simulink model "gm_sampleModel1636_4_sub"  (R2023a)
settings: Solver=VariableStepAuto  StartTime=0.0  StopTime=10.0  RelTol=1e-3
libraries: hdlsllib x4, simulink x1
settings Model: Creator=user1  LastModifiedBy=user1
settings OptimizationCC: BlockReduction=off  ConditionallyExecuteInputs=off
settings DebuggingCC: InheritedTsInSrcMsg=none

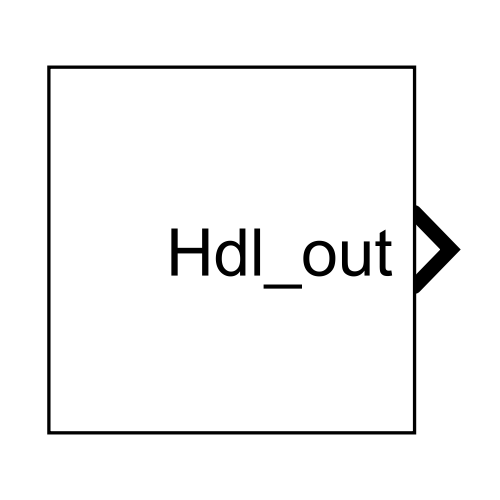
[thumbnail: Simulink's stored preview of the top-level diagram]
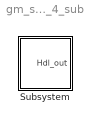
== system gm_sampleModel1636_4_sub ==
  Subsystem : Subsystem

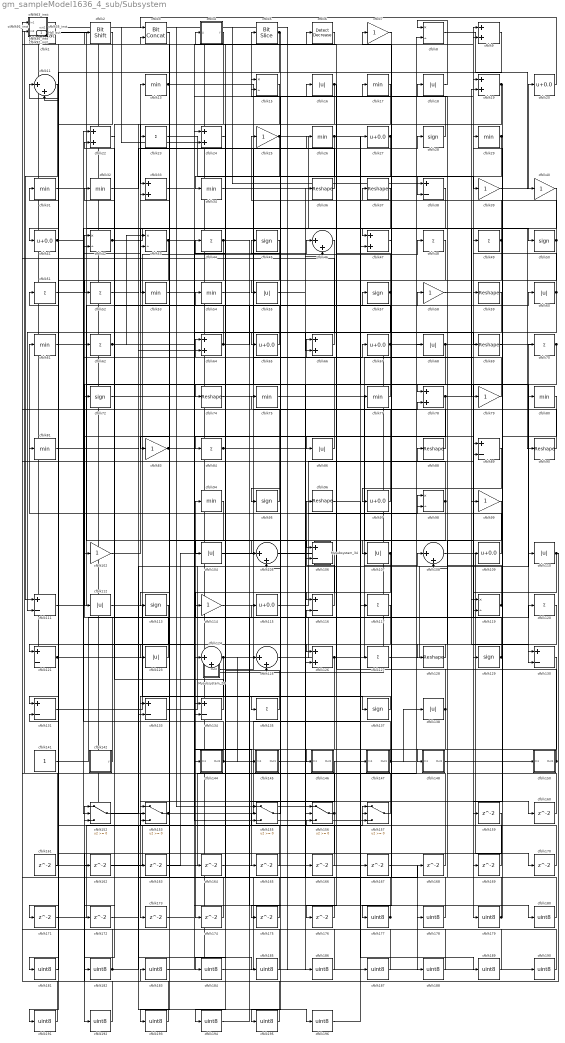
== system gm_sampleModel1636_4_sub/Subsystem ==
  Mysubsystem_20 : Subsystem
  Mysubsystem_34 : Subsystem
  cfblk1 : hdlsllib/Logic and Bit Operations/Bit Concat  numInputs=2
  cfblk101_inst : Subsystem
  cfblk{7,25,39..40,58,79,83,99,102,114} (10 alike) : Gain  OutDataTypeStr=uint8
  cfblk{16,18,55,60,68,86,104,107,110,112,123,138} (12 alike) : Abs  OutDataTypeStr=uint8  SaturateOnIntegerOverflow=off
  cfblk{11,46,105,108,124..125} (6 alike) : Sum  Inputs=|++  OutDataTypeStr=uint8
  cfblk{38,89,106,111,116,121,130..131,133..134} (10 alike) : Sum  Inputs=+-  OutDataTypeStr=uint8
  cfblk{20,27,41,65,67,97,109,115} (8 alike) : Bias  Bias=0.0  SaturateOnIntegerOverflow=off
  cfblk{28,45,50,57,72,95,113,129,137} (9 alike) : Signum
  cfblk{23,44,48..49,51..52,62,70,84,117,120,127,135} (13 alike) : Sum  Inputs=+  OutDataTypeStr=uint8
  cfblk{8,15,42..43,98,119} (6 alike) : Product  Inputs=*/  OutDataTypeStr=uint8  RndMeth=Zero  SaturateOnIntegerOverflow=on
  cfblk122_inst : Subsystem
  cfblk{9,19,22,24,33,47,64,66,78,126} (10 alike) : Sum  OutDataTypeStr=uint8
  cfblk{36..37,59,69,74,88,90,96,128} (9 alike) : Reshape
  cfblk12_inst : Subsystem
  cfblk{13,17,26,29,31..32,34,53..54,61,75,77,80..81,94} (15 alike) : MinMax  OutDataTypeStr=uint8
  cfblk141 : Constant  OutDataTypeStr=uint8  SampleTime=-1
  cfblk142 : Subsystem  mask(Counter Free-Running){NumBits=double(16), tsamp=double(-1)}
      mask prompts: NumBits "Simulink:masks:NumberOfBits_MP"; tsamp "Simulink:masks:SampleTime_MP"
      mask help: Simulink:masks:CounterFreeRunning_MD
  cfblk144 : Subsystem
  cfblk145 : Subsystem
  cfblk146 : Subsystem
  cfblk147 : Subsystem
  cfblk148 : Subsystem
  cfblk150 : Subsystem
  cfblk{152..153,155..157} (5 alike) : Switch  OutDataTypeStr=uint8  SaturateOnIntegerOverflow=off  InputSameDT=off
  cfblk{159..176} (18 alike) : Delay  SampleTime=1
  cfblk{177..196} (20 alike) : DataTypeConversion  OutDataTypeStr=uint8  SaturateOnIntegerOverflow=off  RndMeth=Floor
  cfblk2 : hdlsllib/Logic and Bit Operations/Bit Shift  mode=Shift Left Logical  N=0
  cfblk3 : hdlsllib/Logic and Bit Operations/Bit Concat  numInputs=2
  cfblk30_inst : Subsystem
  cfblk35_inst : Subsystem
  cfblk4 : Subsystem  mask(Detect Rise Nonnegative){vinit=double(0), InputProcessing=Elements as channels (sample based), OutDataTypeStr=uint8}
      mask prompts: vinit "Simulink:masks:InitialCondition_MP"; InputProcessing "Simulink:masks:InputProcessing_MP"; OutDataTypeStr "Simulink:masks:OutputDataType_MP"
      mask help: Simulink:masks:DetectRiseNonnegative_MD
      mask init:
      | InputProcessing = 'Elements as channels (sample based)';
      | OutDataTypeStr = 'uint8';
      | vinit = double(0);
      mask TypeOptions InputProcessing: Simulink:masks:ColumnsAsChannelsFrameBased | Simulink:masks:ElementsAsChannelsSampleBased
      mask TypeOptions OutDataTypeStr: Simulink:masks:uint8 | Simulink:masks:boolean
      mask Display: fprintf('U >= 0\n&  NOT\nU/z >= 0')
  cfblk5 : hdlsllib/Logic and Bit Operations/Bit Slice  lidx=7  ridx=0
  cfblk6 : simulink/Logic and Bit Operations/Detect Decrease  vinit=0.0  OutDataTypeStr=uint8
      settings: LibrarySourceBlock=|
      | hdlsllib/Logic and Bit
      | Operations/Detect
      | Decrease
  cfblk63_inst : Subsystem
  cfblk91_inst : Subsystem
  cfblk92_inst : Subsystem
  Hdl_out : Outport  OutDataTypeStr=uint8  SampleTime=1
  wires:
  Mysubsystem_20/1(Out2) -> cfblk78/2
  Mysubsystem_34/1(Out1) -> cfblk161/1
  cfblk1/1 -> cfblk179/1
  cfblk101_inst/1(out1) -> cfblk190/1
  cfblk102/1 -> cfblk13/1
  cfblk104/1 -> cfblk67/1
  cfblk105/1 -> cfblk88/1
  cfblk106/1 -> cfblk174/1
  cfblk107/1 -> cfblk134/2, cfblk144/1(In1)
  cfblk108/1 -> cfblk170/1
  cfblk109/1 -> cfblk61/1
  cfblk11/1 -> cfblk111/1
  cfblk110/1 -> cfblk183/1, cfblk169/1
  cfblk111/1 -> cfblk54/1
  cfblk112/1 -> cfblk135/1
  cfblk113/1 -> cfblk191/1
  cfblk114/1 -> cfblk28/1
  cfblk115/1 -> cfblk98/1
  cfblk116/1 -> cfblk96/1
  cfblk117/1 -> cfblk195/1
  cfblk119/1 -> cfblk66/1, cfblk75/1
  cfblk12_inst/1(out1) -> cfblk187/1
  cfblk120/1 -> cfblk193/1
  cfblk121/1 -> cfblk137/1, cfblk48/1
  cfblk122_inst/1(out1) -> cfblk156/1, cfblk167/1
  cfblk123/1 -> cfblk42/1
  cfblk124/1 -> cfblk116/2, cfblk173/1
  cfblk125/1 -> cfblk68/1
  cfblk126/1 -> cfblk9/1, cfblk184/1, cfblk108/1
  cfblk127/1 -> cfblk70/1
  cfblk128/1 -> cfblk121/1
  cfblk129/1 -> cfblk59/1, cfblk94/1
  cfblk13/1 -> cfblk130/2, cfblk166/1
  cfblk130/1 -> cfblk148/1(In1)
  cfblk131/1 -> cfblk58/1
  cfblk133/1 -> cfblk110/1
  cfblk134/1 -> cfblk22/2
  cfblk135/1 -> cfblk44/1
  cfblk137/1 -> cfblk133/1
  cfblk138/1 -> cfblk165/1, cfblk6/1
  cfblk141/1 -> cfblk27/1
  cfblk142/1(y) -> cfblk42/2
  cfblk144/1(Out1) -> cfblk22/1, cfblk125/1
  cfblk145/1(Out1) -> cfblk186/1
  cfblk146/1(Out1) -> cfblk153/1
  cfblk147/1(Out1) -> cfblk89/2, cfblk138/1, cfblk4/1(U)
  cfblk148/1(Out1) -> cfblk150/1(In1)
  cfblk15/1 -> cfblk33/1
  cfblk150/1(Out1) -> cfblk37/1, cfblk17/1
  cfblk152/1 -> Mysubsystem_34/1(In1)
  cfblk153/1 -> cfblk47/2, Hdl_out/1
  cfblk155/1 -> cfblk115/1
  cfblk156/1 -> cfblk192/1, cfblk31/1
  cfblk157/1 -> cfblk45/1
  cfblk159/1 -> cfblk181/1
  cfblk16/1 -> cfblk65/1, cfblk133/2, cfblk126/1
  cfblk160/1 -> cfblk98/2
  cfblk161/1 -> cfblk91_inst/2(in2)
  cfblk162/1 -> cfblk155/2
  cfblk163/1 -> cfblk8/2
  cfblk164/1 -> cfblk157/1
  cfblk165/1 -> cfblk153/2
  cfblk166/1 -> cfblk155/1
  cfblk167/1 -> cfblk188/1
  cfblk168/1 -> cfblk63_inst/2(in2)
  cfblk169/1 -> cfblk156/3
  cfblk17/1 -> cfblk84/1
  cfblk170/1 -> cfblk11/1
  cfblk171/1 -> cfblk153/3
  cfblk172/1 -> cfblk157/2
  cfblk173/1 -> cfblk180/1
  cfblk174/1 -> cfblk134/1
  cfblk175/1 -> cfblk131/2
  cfblk176/1 -> cfblk64/1
  cfblk177/1 -> cfblk63_inst/1(in1), cfblk3/2
  cfblk178/1 -> cfblk7/1
  cfblk179/1 -> cfblk108/2, cfblk49/1
  cfblk18/1 -> cfblk8/1
  cfblk180/1 -> cfblk1/1
  cfblk181/1 -> cfblk1/2
  cfblk182/1 -> cfblk92_inst/1(in1), cfblk168/1
  cfblk183/1 -> cfblk46/1
  cfblk184/1 -> cfblk46/2
  cfblk185/1 -> cfblk122_inst/1(in1)
  cfblk186/1 -> cfblk81/1
  cfblk187/1 -> cfblk122_inst/2(in2)
  cfblk188/1 -> cfblk12_inst/1(in1)
  cfblk189/1 -> cfblk12_inst/2(in2)
  cfblk19/1 -> cfblk106/1, cfblk119/2
  cfblk190/1 -> cfblk152/1
  cfblk191/1 -> cfblk101_inst/1(in1)
  cfblk192/1 -> cfblk101_inst/2(in2)
  cfblk193/1 -> cfblk152/3
  cfblk194/1 -> cfblk120/1
  cfblk195/1 -> cfblk91_inst/1(in1)
  cfblk196/1 -> cfblk117/1
  cfblk2/1 -> cfblk41/1
  cfblk20/1 -> cfblk3/1
  cfblk22/1 -> cfblk52/1
  cfblk23/1 -> cfblk39/1
  cfblk24/1 -> cfblk74/1
  cfblk25/1 -> cfblk119/1, cfblk34/1
  cfblk26/1 -> cfblk78/1, cfblk175/1
  cfblk27/1 -> cfblk47/1, cfblk105/1
  cfblk28/1 -> cfblk5/1
  cfblk29/1 -> cfblk38/2, cfblk116/1
  cfblk3/1 -> cfblk113/1
  cfblk30_inst/1(out1) -> cfblk24/2
  cfblk31/1 -> cfblk99/1
  cfblk32/1 -> cfblk26/1
  cfblk33/1 -> cfblk19/1
  cfblk34/1 -> cfblk90/1
  cfblk35_inst/1(out1) -> cfblk121/2, cfblk127/1
  cfblk36/1 -> cfblk23/1
  cfblk37/1 -> cfblk172/1
  cfblk38/1 -> cfblk152/2
  cfblk39/1 -> cfblk20/1
  cfblk4/1(Y) -> cfblk162/1
  cfblk40/1 -> cfblk53/1
  cfblk41/1 -> cfblk86/1, cfblk43/2
  cfblk42/1 -> cfblk50/1, cfblk196/1
  cfblk43/1 -> cfblk69/1, cfblk131/1
  cfblk44/1 -> cfblk156/2, cfblk83/1
  cfblk45/1 -> cfblk123/1
  cfblk46/1 -> cfblk182/1
  cfblk47/1 -> cfblk107/1
  cfblk48/1 -> cfblk194/1
  cfblk49/1 -> cfblk25/1, cfblk146/1(In1)
  cfblk5/1 -> cfblk95/1, cfblk11/2
  cfblk50/1 -> cfblk55/1, cfblk16/1, cfblk15/1
  cfblk51/1 -> cfblk124/1
  cfblk52/1 -> cfblk64/2
  cfblk53/1 -> cfblk155/3
  cfblk54/1 -> cfblk178/1
  cfblk55/1 -> cfblk36/1
  cfblk57/1 -> cfblk2/1, cfblk125/2, cfblk111/2
  cfblk58/1 -> cfblk79/1
  cfblk59/1 -> cfblk164/1
  cfblk6/1 -> cfblk92_inst/2(in2)
  cfblk60/1 -> cfblk66/2, cfblk29/1
  cfblk61/1 -> cfblk106/2
  cfblk62/1 -> cfblk89/1, cfblk43/1
  cfblk63_inst/1(out1) -> cfblk157/3
  cfblk64/1 -> cfblk57/1, cfblk33/2
  cfblk65/1 -> cfblk32/1
  cfblk66/1 -> cfblk30_inst/2(in2)
  cfblk67/1 -> cfblk112/1, cfblk15/2
  cfblk68/1 -> cfblk105/2, cfblk176/1
  cfblk69/1 -> cfblk159/1
  cfblk7/1 -> cfblk177/1
  cfblk70/1 -> cfblk124/2, cfblk102/1
  cfblk72/1 -> cfblk80/1
  cfblk74/1 -> cfblk160/1
  cfblk75/1 -> cfblk109/1
  cfblk77/1 -> cfblk72/1
  cfblk78/1 -> cfblk19/2, cfblk130/1, cfblk104/1
  cfblk79/1 -> cfblk18/1
  cfblk8/1 -> cfblk40/1
  cfblk80/1 -> cfblk129/1
  cfblk81/1 -> cfblk185/1
  cfblk83/1 -> cfblk9/2, cfblk145/1(In1)
  cfblk84/1 -> cfblk60/1, cfblk126/2
  cfblk86/1 -> cfblk62/1
  cfblk88/1 -> cfblk24/1
  cfblk89/1 -> cfblk97/1
  cfblk9/1 -> cfblk171/1
  cfblk90/1 -> cfblk51/1
  cfblk91_inst/1(out1) -> cfblk38/1, cfblk147/1(In1)
  cfblk92_inst/1(out1) -> cfblk77/1
  cfblk94/1 -> cfblk163/1
  cfblk95/1 -> cfblk30_inst/1(in1)
  cfblk96/1 -> cfblk189/1
  cfblk97/1 -> cfblk35_inst/1(in1)
  cfblk98/1 -> cfblk35_inst/2(in2), cfblk114/1
  cfblk99/1 -> cfblk128/1

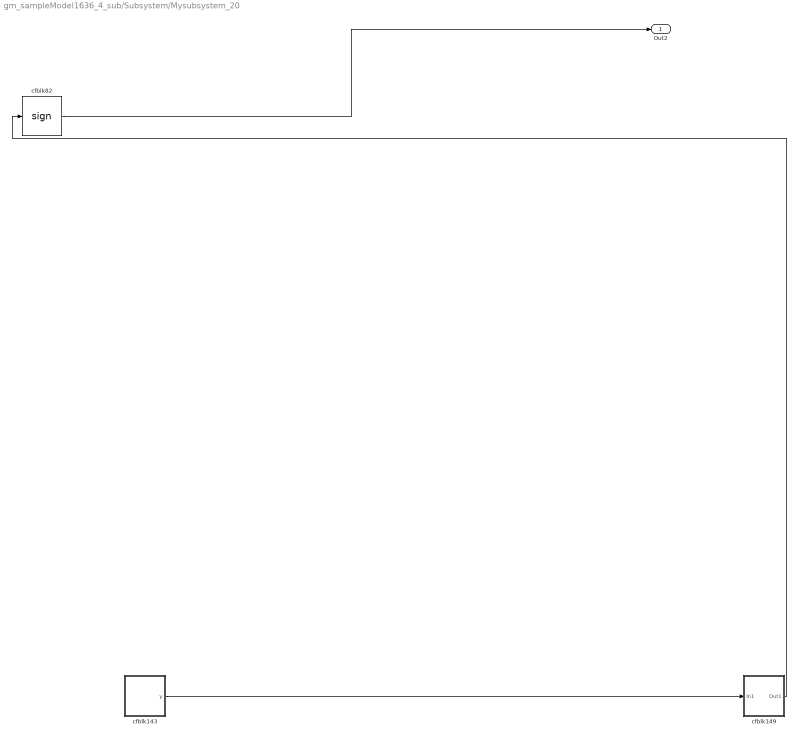
== system gm_sampleModel1636_4_sub/Subsystem/Mysubsystem_20 ==
  cfblk143 : Subsystem  mask(Counter Limited){uplimit=double(7), tsamp=double(-1)}
      mask prompts: uplimit "Simulink:masks:UpperLimit_MP"; tsamp "Simulink:masks:SampleTime_MP"
      mask help: Simulink:masks:CounterLimited_MD
      mask init:
      | nbits = double(8);
      | tsamp = double(-1);
      | uplimit = double(7);
  cfblk149 : Subsystem
  cfblk82 : Signum
  Out2 : Outport  SampleTime=1
  wires:
  cfblk143/1(y) -> cfblk149/1(In1)
  cfblk149/1(Out1) -> cfblk82/1
  cfblk82/1 -> Out2/1

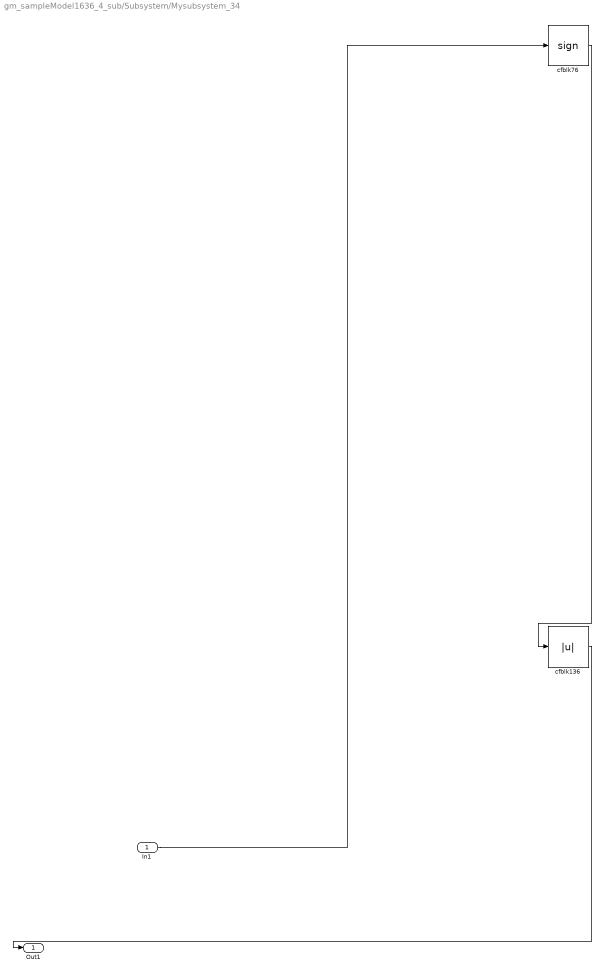
== system gm_sampleModel1636_4_sub/Subsystem/Mysubsystem_34 ==
  In1 : Inport  OutDataTypeStr=uint8  PortDimensions=1  SampleTime=1
  cfblk136 : Abs  SaturateOnIntegerOverflow=off
  cfblk76 : Signum
  Out1 : Outport  SampleTime=1
  wires:
  In1/1 -> cfblk76/1
  cfblk136/1 -> Out1/1
  cfblk76/1 -> cfblk136/1

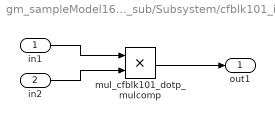
== system gm_sampleModel1636_4_sub/Subsystem/cfblk101_inst ==
  in1 : Inport  OutDataTypeStr=uint8  SampleTime=1
  in2 : Inport  Port=2  OutDataTypeStr=uint8  SampleTime=1
  mul_cfblk101_dotp_mulcomp : Product  Inputs=**  OutDataTypeStr=uint8  SampleTime=1
  out1 : Outport  OutDataTypeStr=uint8  SampleTime=1
  wires:
  in1/1 -> mul_cfblk101_dotp_mulcomp/1
  in2/1 -> mul_cfblk101_dotp_mulcomp/2
  mul_cfblk101_dotp_mulcomp/1 -> out1/1

== system gm_sampleModel1636_4_sub/Subsystem/cfblk122_inst ==
  in1 : Inport  OutDataTypeStr=uint8  SampleTime=1
  in2 : Inport  Port=2  OutDataTypeStr=uint8  SampleTime=1
  mul_cfblk122_dotp_mulcomp : Product  Inputs=**  OutDataTypeStr=uint8  SampleTime=1
  out1 : Outport  OutDataTypeStr=uint8  SampleTime=1
  wires:
  in1/1 -> mul_cfblk122_dotp_mulcomp/1
  in2/1 -> mul_cfblk122_dotp_mulcomp/2
  mul_cfblk122_dotp_mulcomp/1 -> out1/1

== system gm_sampleModel1636_4_sub/Subsystem/cfblk12_inst ==
  in1 : Inport  OutDataTypeStr=uint8  SampleTime=1
  in2 : Inport  Port=2  OutDataTypeStr=uint8  SampleTime=1
  mul_cfblk12_dotp_mulcomp : Product  Inputs=**  OutDataTypeStr=uint8  SampleTime=1
  out1 : Outport  OutDataTypeStr=uint8  SampleTime=1
  wires:
  in1/1 -> mul_cfblk12_dotp_mulcomp/1
  in2/1 -> mul_cfblk12_dotp_mulcomp/2
  mul_cfblk12_dotp_mulcomp/1 -> out1/1

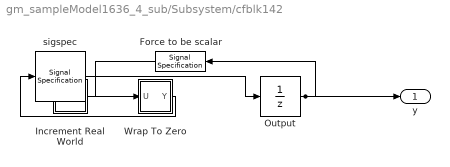
== system gm_sampleModel1636_4_sub/Subsystem/cfblk142 ==
  Force to be scalar : SignalSpecification  DisableCoverage=on  Dimensions=1
  Increment Real World : Subsystem  mask(Real World Value Increment){}
      mask help: Simulink:masks:RealWorldValueIncrement_MD
      mask Display: disp('V++')
  Output : UnitDelay  InitialCondition=0.0  SampleTime=tsamp  HasFrameUpgradeWarning=on
  Wrap To Zero : Subsystem  mask(Wrap To Zero){Threshold=double(65535)}
      mask prompts: Threshold "Simulink:masks:Threshold_MP"
      mask help: Simulink:masks:WrapToZero_MD
  sigspec : SignalSpecification  OutDataTypeStr=uint16  Dimensions=1
  y : Outport  SampleTime=1
  wires:
  Force to be scalar/1 -> Increment Real World/1(u)
  Increment Real World/1(y) -> Wrap To Zero/1(U)
  Output/1 -> Force to be scalar/1, y/1
  Wrap To Zero/1(Y) -> sigspec/1
  sigspec/1 -> Output/1

== system gm_sampleModel1636_4_sub/Subsystem/cfblk144 ==
  In1 : Inport  OutDataTypeStr=uint8  PortDimensions=1  SampleTime=1
  Out1 : Outport  SampleTime=1
  wires:
  In1/1 -> Out1/1

== system gm_sampleModel1636_4_sub/Subsystem/cfblk145 ==
  In1 : Inport  OutDataTypeStr=uint8  PortDimensions=1  SampleTime=1
  Out1 : Outport  SampleTime=1
  wires:
  In1/1 -> Out1/1

== system gm_sampleModel1636_4_sub/Subsystem/cfblk146 ==
  In1 : Inport  OutDataTypeStr=uint8  PortDimensions=1  SampleTime=1
  Out1 : Outport  SampleTime=1
  wires:
  In1/1 -> Out1/1

== system gm_sampleModel1636_4_sub/Subsystem/cfblk147 ==
  In1 : Inport  OutDataTypeStr=uint8  PortDimensions=1  SampleTime=1
  Out1 : Outport  SampleTime=1
  wires:
  In1/1 -> Out1/1

== system gm_sampleModel1636_4_sub/Subsystem/cfblk148 ==
  In1 : Inport  OutDataTypeStr=uint8  PortDimensions=1  SampleTime=1
  Out1 : Outport  SampleTime=1
  wires:
  In1/1 -> Out1/1

== system gm_sampleModel1636_4_sub/Subsystem/cfblk150 ==
  In1 : Inport  OutDataTypeStr=uint8  PortDimensions=1  SampleTime=1
  Out1 : Outport  SampleTime=1
  wires:
  In1/1 -> Out1/1

== system gm_sampleModel1636_4_sub/Subsystem/cfblk30_inst ==
  in1 : Inport  OutDataTypeStr=uint8  SampleTime=1
  in2 : Inport  Port=2  OutDataTypeStr=uint8  SampleTime=1
  mul_cfblk30_dotp_mulcomp : Product  Inputs=**  OutDataTypeStr=uint8  SampleTime=1
  out1 : Outport  OutDataTypeStr=uint8  SampleTime=1
  wires:
  in1/1 -> mul_cfblk30_dotp_mulcomp/1
  in2/1 -> mul_cfblk30_dotp_mulcomp/2
  mul_cfblk30_dotp_mulcomp/1 -> out1/1

== system gm_sampleModel1636_4_sub/Subsystem/cfblk35_inst ==
  in1 : Inport  OutDataTypeStr=uint8  SampleTime=1
  in2 : Inport  Port=2  OutDataTypeStr=uint8  SampleTime=1
  mul_cfblk35_dotp_mulcomp : Product  Inputs=**  OutDataTypeStr=uint8  SampleTime=1
  out1 : Outport  OutDataTypeStr=uint8  SampleTime=1
  wires:
  in1/1 -> mul_cfblk35_dotp_mulcomp/1
  in2/1 -> mul_cfblk35_dotp_mulcomp/2
  mul_cfblk35_dotp_mulcomp/1 -> out1/1

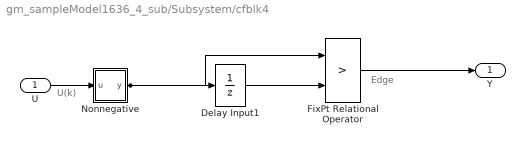
== system gm_sampleModel1636_4_sub/Subsystem/cfblk4 ==
  note: U(k)
  note: Edge
  U : Inport  OutDataTypeStr=uint8  SampleTime=1
  Delay Input1 : UnitDelay  Description=Store in Global RAM  DisableCoverage=on  InitialCondition=vinit  SampleTime=-1  HasFrameUpgradeWarning=on
  FixPt Relational Operator : RelationalOperator  Operator=>  OutDataTypeStr=fixdt(0, 8)  ZeroCross=off  InputSameDT=off
  Nonnegative : Subsystem  mask(Compare To Zero){relop=>=, OutDataTypeStr=boolean, ZeroCross=off}
      mask prompts: relop "Simulink:masks:Operator_MP"; OutDataTypeStr "Simulink:masks:OutputDataType_MP"; ZeroCross "Simulink:masks:EnableZerocrossingDetection_MP"
      mask help: Simulink:masks:CompareToZero_MD
      mask init:
      | OutDataTypeStr = 'boolean';
      | ZeroCross = 'off';
      | blkName = 'sampleModel1636_4_sub/Subsystem/cfblk4/Nonnegative';
      | relop = '>=';
      | setValue = 'boolean';
      mask TypeOptions relop: == | ~= | < | <= | >= | >
      mask TypeOptions OutDataTypeStr: Simulink:masks:uint8 | Simulink:masks:boolean
      mask Callback ZeroCross: sl('zeroCrossEnable', gcbh);
      mask Display: disp([relop,' 0'])
  Y : Outport  SampleTime=1
  wires:
  U/1 -> Nonnegative/1(u)
  Delay Input1/1 -> FixPt Relational Operator/2
  FixPt Relational Operator/1 -> Y/1
  Nonnegative/1(y) -> FixPt Relational Operator/1, Delay Input1/1

== system gm_sampleModel1636_4_sub/Subsystem/cfblk63_inst ==
  in1 : Inport  OutDataTypeStr=uint8  SampleTime=1
  in2 : Inport  Port=2  OutDataTypeStr=uint8  SampleTime=1
  mul_cfblk63_dotp_mulcomp : Product  Inputs=**  OutDataTypeStr=uint8  SampleTime=1
  out1 : Outport  OutDataTypeStr=uint8  SampleTime=1
  wires:
  in1/1 -> mul_cfblk63_dotp_mulcomp/1
  in2/1 -> mul_cfblk63_dotp_mulcomp/2
  mul_cfblk63_dotp_mulcomp/1 -> out1/1

== system gm_sampleModel1636_4_sub/Subsystem/cfblk91_inst ==
  in1 : Inport  OutDataTypeStr=uint8  SampleTime=1
  in2 : Inport  Port=2  OutDataTypeStr=uint8  SampleTime=1
  mul_cfblk91_dotp_mulcomp : Product  Inputs=**  OutDataTypeStr=uint8  SampleTime=1
  out1 : Outport  OutDataTypeStr=uint8  SampleTime=1
  wires:
  in1/1 -> mul_cfblk91_dotp_mulcomp/1
  in2/1 -> mul_cfblk91_dotp_mulcomp/2
  mul_cfblk91_dotp_mulcomp/1 -> out1/1

== system gm_sampleModel1636_4_sub/Subsystem/cfblk92_inst ==
  in1 : Inport  OutDataTypeStr=uint8  SampleTime=1
  in2 : Inport  Port=2  OutDataTypeStr=uint8  SampleTime=1
  mul_cfblk92_dotp_mulcomp : Product  Inputs=**  OutDataTypeStr=uint8  SampleTime=1
  out1 : Outport  OutDataTypeStr=uint8  SampleTime=1
  wires:
  in1/1 -> mul_cfblk92_dotp_mulcomp/1
  in2/1 -> mul_cfblk92_dotp_mulcomp/2
  mul_cfblk92_dotp_mulcomp/1 -> out1/1

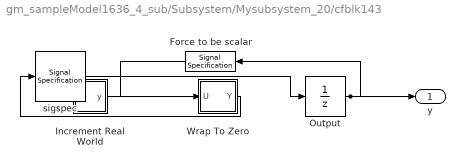
== system gm_sampleModel1636_4_sub/Subsystem/Mysubsystem_20/cfblk143 ==
  Force to be scalar : SignalSpecification  DisableCoverage=on  Dimensions=1
  Increment Real World : Subsystem  mask(Real World Value Increment){}
      mask help: Simulink:masks:RealWorldValueIncrement_MD
      mask Display: disp('V++')
  Output : UnitDelay  InitialCondition=0.0  SampleTime=tsamp  HasFrameUpgradeWarning=on
  Wrap To Zero : Subsystem  mask(Wrap To Zero){Threshold=double(7)}
      mask prompts: Threshold "Simulink:masks:Threshold_MP"
      mask help: Simulink:masks:WrapToZero_MD
  sigspec : SignalSpecification  OutDataTypeStr=uint8  Dimensions=1
  y : Outport  SampleTime=1
  wires:
  Force to be scalar/1 -> Increment Real World/1(u)
  Increment Real World/1(y) -> Wrap To Zero/1(U)
  Output/1 -> Force to be scalar/1, y/1
  Wrap To Zero/1(Y) -> sigspec/1
  sigspec/1 -> Output/1

== system gm_sampleModel1636_4_sub/Subsystem/Mysubsystem_20/cfblk149 ==
  In1 : Inport  OutDataTypeStr=uint8  PortDimensions=1  SampleTime=1
  Out1 : Outport  SampleTime=1
  wires:
  In1/1 -> Out1/1

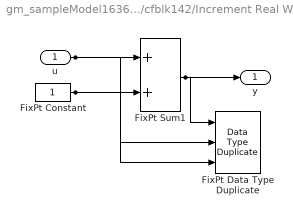
== system gm_sampleModel1636_4_sub/Subsystem/cfblk142/Increment Real World ==
  u : Inport  OutDataTypeStr=uint16  SampleTime=1
  FixPt Constant : Constant  DisableCoverage=on  OutDataTypeStr=Inherit: Inherit via back propagation  SampleTime=-1
  FixPt Data Type Duplicate : DataTypeDuplicate  DisableCoverage=on  NumInputPorts=3
  FixPt Sum1 : Sum  InputSameDT=on  OutDataTypeStr=Inherit: Inherit via back propagation  LockScale=on
  y : Outport  SampleTime=1
  wires:
  u/1 -> FixPt Sum1/1, FixPt Data Type Duplicate/2
  FixPt Constant/1 -> FixPt Sum1/2, FixPt Data Type Duplicate/3
  FixPt Sum1/1 -> FixPt Data Type Duplicate/1, y/1

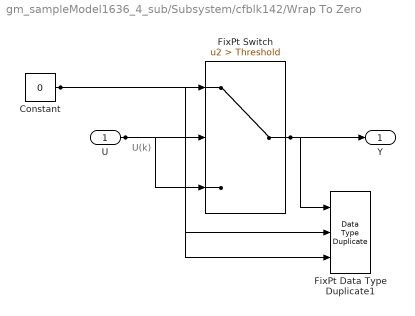
== system gm_sampleModel1636_4_sub/Subsystem/cfblk142/Wrap To Zero ==
  note: U(k)
  U : Inport  OutDataTypeStr=uint16  SampleTime=1
  Constant : Constant  DisableCoverage=on  Value=0  OutDataTypeStr=Inherit: Inherit via back propagation  SampleTime=-1
  FixPt Data Type Duplicate1 : DataTypeDuplicate  DisableCoverage=on  NumInputPorts=3
  FixPt Switch : Switch  Criteria=u2 > Threshold  Threshold=Threshold  OutDataTypeStr=Inherit: Inherit via back propagation  ZeroCross=off  SaturateOnIntegerOverflow=off  InputSameDT=off
  Y : Outport  SampleTime=1
  wires:
  U/1 -> FixPt Switch/3, FixPt Switch/2, FixPt Data Type Duplicate1/2
  Constant/1 -> FixPt Switch/1, FixPt Data Type Duplicate1/3
  FixPt Switch/1 -> FixPt Data Type Duplicate1/1, Y/1

== system gm_sampleModel1636_4_sub/Subsystem/cfblk4/Nonnegative ==
  u : Inport  OutDataTypeStr=uint8  SampleTime=1
  Compare : RelationalOperator  OutDataTypeStr=boolean  ZeroCross=off
  Constant : Constant  DisableCoverage=on  Value=0  OutDataTypeStr=Inherit: Inherit via back propagation  SampleTime=-1  PreserveConstantTs=on
  y : Outport  SampleTime=1
  wires:
  u/1 -> Compare/1
  Compare/1 -> y/1
  Constant/1 -> Compare/2

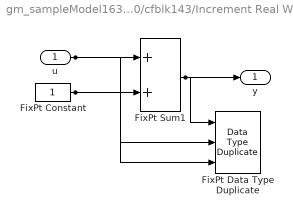
== system gm_sampleModel1636_4_sub/Subsystem/Mysubsystem_20/cfblk143/Increment Real World ==
  u : Inport  OutDataTypeStr=uint8  SampleTime=1
  FixPt Constant : Constant  DisableCoverage=on  OutDataTypeStr=Inherit: Inherit via back propagation  SampleTime=-1
  FixPt Data Type Duplicate : DataTypeDuplicate  DisableCoverage=on  NumInputPorts=3
  FixPt Sum1 : Sum  InputSameDT=on  OutDataTypeStr=Inherit: Inherit via back propagation  LockScale=on
  y : Outport  SampleTime=1
  wires:
  u/1 -> FixPt Sum1/1, FixPt Data Type Duplicate/2
  FixPt Constant/1 -> FixPt Sum1/2, FixPt Data Type Duplicate/3
  FixPt Sum1/1 -> FixPt Data Type Duplicate/1, y/1

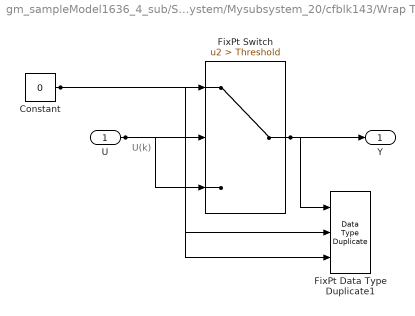
== system gm_sampleModel1636_4_sub/Subsystem/Mysubsystem_20/cfblk143/Wrap To Zero ==
  note: U(k)
  U : Inport  OutDataTypeStr=uint8  SampleTime=1
  Constant : Constant  DisableCoverage=on  Value=0  OutDataTypeStr=Inherit: Inherit via back propagation  SampleTime=-1
  FixPt Data Type Duplicate1 : DataTypeDuplicate  DisableCoverage=on  NumInputPorts=3
  FixPt Switch : Switch  Criteria=u2 > Threshold  Threshold=Threshold  OutDataTypeStr=Inherit: Inherit via back propagation  ZeroCross=off  SaturateOnIntegerOverflow=off  InputSameDT=off
  Y : Outport  SampleTime=1
  wires:
  U/1 -> FixPt Switch/3, FixPt Switch/2, FixPt Data Type Duplicate1/2
  Constant/1 -> FixPt Switch/1, FixPt Data Type Duplicate1/3
  FixPt Switch/1 -> FixPt Data Type Duplicate1/1, Y/1
